simulink model "DCmotor"  (R2016a)
settings: Solver=ode23t  StartTime=0.0  StopTime=10.0  RelTol=1e-3  AbsTol=1e-3
libraries: fl_lib x12, nesl_utility x3
settings Model: Creator=STF2972  LastModifiedBy=stf2972
settings GRTTargetCC: GeneratePreprocessorConditionals=Use local settings
settings SimscapeCC: SimscapeLogType=all  SimscapeLogDataHistory=10000

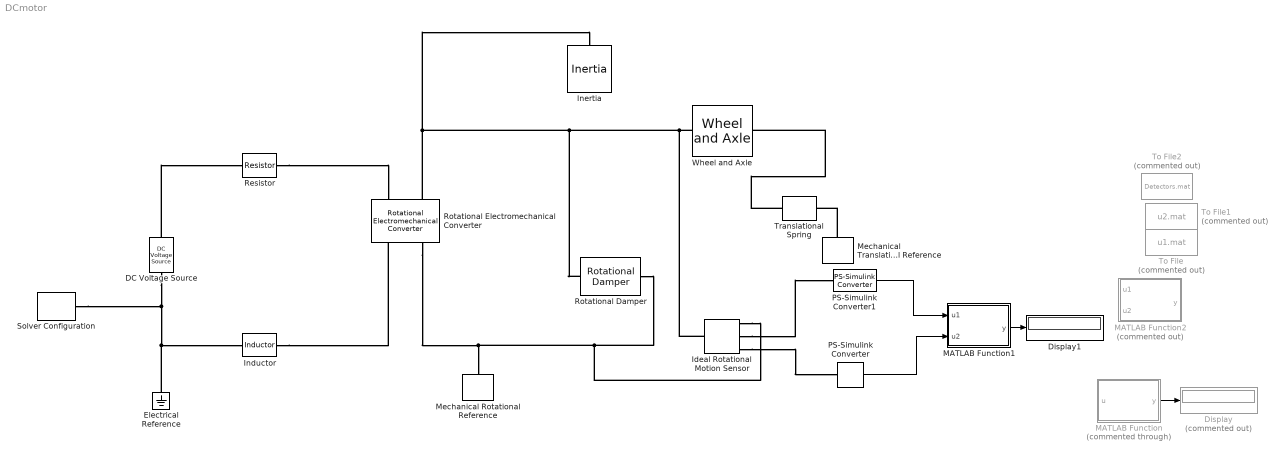
== system DCmotor ==
  DC Voltage Source : fl_lib/Electrical/Electrical Sources/DC Voltage Source  v0=5 V
  Display : Display  Commented=on
  Display1 : Display
  Electrical Reference : fl_lib/Electrical/Electrical Elements/Electrical Reference
  Ideal Rotational Motion Sensor : fl_lib/Mechanical/Mechanical Sensors/Ideal Rotational Motion Sensor  offset=0 rad
  Inductor : fl_lib/Electrical/Electrical Elements/Inductor  l=1e-6 H  r=0 Ohm  g=1e-9 1/Ohm  i_specify=off  i_priority=None  i=0 A  v_specify=off  v_priority=None  v=0 V  i_L_specify=off  i_L_priority=High  i_L=0 A
  Inertia : fl_lib/Mechanical/Rotational Elements/Inertia  inertia=0.02 kg*m^2  w_specify=off  w_priority=High  w=0 rad/s  t_specify=off  t_priority=None  t=0 N*m
  MATLAB Function : MATLAB Function  Commented=through  TreatAsAtomicUnit=on
  MATLAB Function1 : MATLAB Function  TreatAsAtomicUnit=on
  MATLAB Function2 : MATLAB Function  Commented=on  TreatAsAtomicUnit=on
  Mechanical Rotational Reference : fl_lib/Mechanical/Rotational Elements/Mechanical Rotational Reference
  Mechanical Translational Reference : fl_lib/Mechanical/Translational Elements/Mechanical Translational Reference
  PS-Simulink Converter : nesl_utility/PS-Simulink Converter  PhysicalDomain=network_engine_domain  SubClassName=ps_output  LeftPortType=input  RightPortType=output  PseudoPeriodic=off  Frequencies=[]  Unit=deg  AffineConversion=off
  PS-Simulink Converter1 : nesl_utility/PS-Simulink Converter  PhysicalDomain=network_engine_domain  SubClassName=ps_output  LeftPortType=input  RightPortType=output  PseudoPeriodic=off  Frequencies=[]  Unit=1  AffineConversion=off
  Resistor : fl_lib/Electrical/Electrical Elements/Resistor  R=1 Ohm  i_specify=off  i_priority=None  i=0 A  v_specify=off  v_priority=None  v=0 V
  Rotational Electromechanical Converter : fl_lib/Electrical/Electrical Elements/Rotational Electromechanical Converter  K=0.1 V/(rad/s)  i_specify=off  i_priority=None  i=0 A  v_specify=off  v_priority=None  v=0 V  t_specify=off  t_priority=None  t=0 N*m  w_specify=off  w_priority=None  w=0 rad/s
  Rotational Damper : fl_lib/Mechanical/Rotational Elements/Rotational Damper  D=0.2 N*m/(rad/s)  w_specify=off  w_priority=None  w=0 rad/s  t_specify=off  t_priority=None  t=0 N*m
  Solver Configuration : nesl_utility/Solver Configuration  PhysicalDomain=network_engine_domain  SubClassName=solver  LeftPortType=input  RightPortType=generic  Accelerate=off  Tones=[]  Harmonics=[]  SimulateNoise=off  Profile=off  UseLocalSampling=off  EnableSwitchedLinearOptims=on  FrequencyDomain=off  UseCCode=off  RelTol=0.001  AbsTol=1e-06  MinStep=1e-09  ToWorkspace=off  RevertToSquareIcSolve=off  NumHomotopyIterations=100  PhasorMode=off  PhasorModeNumHarmonics=1  OverrideAbsTol=off  DoDC=off  ResidualTolerance=1e-09  UseLocalSolver=off  LocalSolverChoice=NE_BACKWARD_EULER_ADVANCER  LocalSolverSampleTime=0.001  DoFixedCost=off  MaxNonlinIter=3  MaxModeIter=2  LinearAlgebra=Sparse  DelaysMemoryBudget=1024  AutomaticFiltering=on  FilteringTimeConstant=0.001
  To File : ToFile  Commented=on  Filename=u1.mat  MatrixName=u_1
  To File1 : ToFile  Commented=on  Filename=u2.mat  MatrixName=u_2
  To File2 : ToFile  Commented=on  Filename=Detectors.mat  MatrixName=detectorSet
  Translational Spring : fl_lib/Mechanical/Translational Elements/Translational Spring  spr_rate=1000 N/m  v_specify=off  v_priority=None  v=0 m/s  f_specify=off  f_priority=None  f=0 N  x_specify=off  x_priority=High  x=0 m
  Wheel and Axle : fl_lib/Mechanical/Mechanisms/Wheel and Axle  R=0.03 m  or=1  t_specify=off  t_priority=None  t=0 N*m  f_specify=off  f_priority=None  f=0 N
  wires:
  PS-Simulink Converter/1 -> MATLAB Function1/2(u2)
  PS-Simulink Converter1/1 -> MATLAB Function1/1(u1)
  MATLAB Function/1(y) -> Display/1
  MATLAB Function1/1(y) -> Display1/1
  connections:
  DC Voltage Source/LConn1 -- Resistor/LConn1
  Resistor/RConn1 -- Rotational Electromechanical Converter/LConn1
  DC Voltage Source/RConn1 -- Solver Configuration/RConn1 -- Electrical Reference/LConn1 -- Inductor/LConn1
  Inductor/RConn1 -- Rotational Electromechanical Converter/RConn1
  Rotational Electromechanical Converter/RConn2 -- Ideal Rotational Motion Sensor/RConn1 -- Rotational Damper/RConn1 -- Mechanical Rotational Reference/LConn1
  Rotational Electromechanical Converter/LConn2 -- Ideal Rotational Motion Sensor/LConn1 -- Wheel and Axle/LConn1 -- Rotational Damper/LConn1 -- Inertia/LConn1
  Translational Spring/LConn1 -- Wheel and Axle/RConn1
  Mechanical Translational Reference/LConn1 -- Translational Spring/RConn1
  Ideal Rotational Motion Sensor/RConn3 -- PS-Simulink Converter/LConn1
  Ideal Rotational Motion Sensor/RConn2 -- PS-Simulink Converter1/LConn1

== matlab function DCmotor/MATLAB Function1 ==
  data: u1 input; u2 input; y output [0..50]

function y = fcn(u1,u2)

%% #codegen
coder.extrinsic('clc');
persistent detSet N  m n rs c_s1 c_s2;




if isempty(rs)
x_1=11.4591559045;
x_2 =11.45915590;


y_1=4e-10; 
y_2=-4e-10; 
%%Distance measures

c_s1 =(x_1+x_2)/2;
c_s2=(y_1+y_2)/2;

if (abs(y_1-y_2)>abs(x_1-x_2))
    rs =abs(x_1-x_2);
else 
    rs =abs(y_1-y_2);
end 
% center of self and the radious 
circle(c_s1, c_s2,rs);
detSet=[c_s1 c_s2 rs];
end
coder.varsize('detSet',[30000000 3]);
% dist_min=0;
% temp_dist=0;
% rDet=0;
%drawCircle(c_s1, c_s2,rs);
%filledCircle([c_s1,c_s2],rs,1000,'r')
%Until N ==m_max
if isempty(N)&&isempty(m)&&isempty(n)
N=0; % count of not self
 
m=0; % count of not self 
p=0.5; % default probability 
n =(max(5/p, 5/(1-p)));
 % sample size/ total number of data
% detected occurances

end

z_alpha =3.49;
 
% Estimated coverage 99% 
%%%% Hyppthesis testing %%%%

% Sample a point 



% %%
% %two dimensional space 
 
 a=u1;
 b =u2;
 


 if(a>0.1 && b>0.1) % to reduce the noise ???     
    if (N<n) % exit criterion 
        n =n+1; % count the sample size
        if(abs (sqrt(((b-c_s2)^2+(a-c_s1)^2))-rs))>rs % Euclidean distance -non self
        %%--------not-self-------
        %%  
        toself =sqrt(((b-c_s2)^2+(a-c_s1)^2))-rs;
        N=N+1; % count (non-self) sample
         
%         if size(detSet,1)==1 % first detector    
%             % addthe first detector to the map
%             c=sqrt(((b-c_s2)^2+(a-c_s1)^2))-rs;
%             detSet=[detSet; [a b c]];
%             %y=detSet;
%             %xlswrite('detectors.xlsx',detSet);
%            
%             circle(a,b,c);                 
%         else
        %find the closest detector
           rDet=0;           
            %finding the minimum distance to the point selected
             dist_min = (b-detSet(1,2))^2+(a-detSet(1,1))^2;
            for j=2: size(detSet,1)                                             
                    temp_dist=(b-detSet(j,2))^2+(a-detSet(j,1))^2;
                    if(temp_dist<dist_min)
                    dist_min=temp_dist;
                    rDet =detSet(j,3);
                    end                              
            end 
                %% check if it is out side of the closest detector                             
            %Check if it is within the raduis of the closest detector
            
        
            %% Covered? yes 
            if rDet>sqrt(dist_min)
                 %% Covered? yes
                m=m+1; % count covered sample
                p =N/n; % probability of not self
                q= 1-p;
                z=m/sqrt(n*p*q)-sqrt(n*p/q); % evaluate z score
                if z<z_alpha % not enough coverage
                    if(N==n) 
                        %% Accept all saved candidates as new detectors
                        N=0;
                        m=0;
                    
                        
                    end 
                else %enough coverage
                    N=n+1; % exist the function
                end 
            else 
                %% Covered? No : save the candidate
                toself
                sqrt(dist_min)
                if toself < sqrt(dist_min)
                    detSet=[detSet; [a b toself]];
                    circle(a,b,toself);
                else
                    detSet=[detSet; [a b sqrt(dist_min)]];
                    circle(a,b,sqrt(dist_min));
                end
               
                detSet
               
           % end    
        end 
        end 
       
    end 
 end 

y =a;
%This assignment writes a 'double' value into a 'embedded.fi {int16}' type. Code generation does not support changing types through assignment. Check preceding assignments or input type specifications for type mismatches.


% 
 

 function circle(x,y,r)
%x and y are the coordinates of the center of the circle
%r is the radius of the circle
%0.01 is the angle step, bigger values will draw the circle faster but
%you might notice imperfections (not very smooth)
ang=0:0.01:2*pi; 
xp=r*cos(ang);
yp=r*sin(ang);
plot(x+xp,y+yp);
hold on

function h = filledCircle(center,r,N,color)
THETA=linspace(0,2*pi,N);
RHO=ones(1,N)*r;
[X,Y] = pol2cart(THETA,RHO);
X=X+center(1);
Y=Y+center(2);
h=fill(X,Y,color);
axis square;

== matlab function DCmotor/MATLAB Function ==
  data: u input; y output [1..2]
function y = fcn(u)
%#codegen
coder.extrinsic('clc');
persistent d n;
if isempty(n)
n=0;
end
% size(d,1)
assert(n<=10000);
coder.varsize('d',[30000000 3]);
b=[u u+1 u+2];
if isempty(d)
    n=1;
d=zeros(n,3);
else 
    n =size(d,1);
    d=[b;d]

end

y = u;

== matlab function DCmotor/MATLAB Function2 ==
  data: u1 input; y output; u2 input
function y = createSelf(u1,u2)
%#codegen
%Boundary aware V-detector system
%% Cross
% Thickness and location of the cross
plot(u1,u2);
%% Triangle
% Size (radius of circumscribed circle)
%% Ring 
% Out and inner radius
%% Stripe 
% Width
%% Intersection 
% cross size and location , circle radius
%% Pentagram 
% side (radius of circumscribed circle)

y = u1;
